simulink model "PR_2_var2"  (R2020b)
settings: Solver=VariableStepAuto  StartTime=0.0  StopTime=50  FixedStep=10^-4  RelTol=1e-3
libraries: simulink x2
settings Model: Creator=SIA  LastModifiedBy=SIA

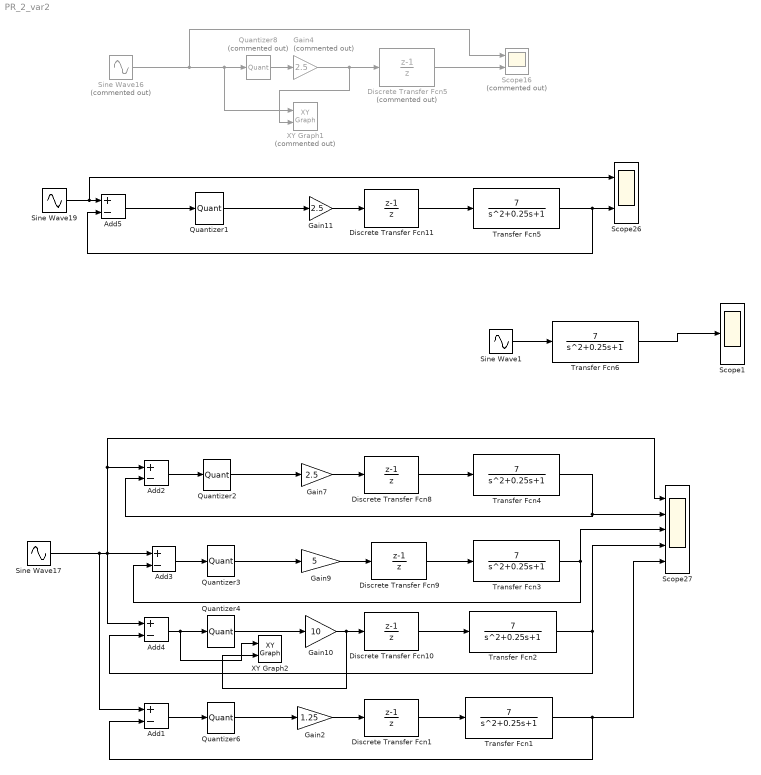
== system PR_2_var2 ==
  Add{1..5} (5 alike) : Sum  Inputs=+-
  Discrete Transfer Fcn{1,8..11} (5 alike) : DiscreteTransferFcn  Numerator=[1 -1]  Denominator=[1 0]  SampleTime=0.05
  Discrete Transfer Fcn5 : DiscreteTransferFcn  Commented=on  Numerator=[1 -1]  Denominator=[1 0]  SampleTime=0.05
  Gain10 : Gain  Gain=10
  Gain11 : Gain  Gain=2.5
  Gain2 : Gain  Gain=1.25
  Gain4 : Gain  Commented=on  Gain=2.5
  Gain7 : Gain  Gain=2.5
  Gain9 : Gain  Gain=5
  Quantizer1 : Quantizer  QuantizationInterval=2
  Quantizer2 : Quantizer  QuantizationInterval=2
  Quantizer3 : Quantizer  QuantizationInterval=1
  Quantizer4 : Quantizer
  Quantizer6 : Quantizer  QuantizationInterval=4
  Quantizer8 : Quantizer  Commented=on  QuantizationInterval=2
  Scope1 : Scope  NumInputPorts=3
  Scope16 : Scope  Commented=on  NumInputPorts=2
  Scope26 : Scope  NumInputPorts=2
  Scope27 : Scope  NumInputPorts=5
  Sine Wave1 : Sin  Amplitude=5*0.5  Frequency=3  SampleTime=0
  Sine Wave16 : Sin  Commented=on  Amplitude=5*1  SampleTime=0
  Sine Wave17 : Sin  Amplitude=5*1  SampleTime=0
  Sine Wave19 : Sin  Amplitude=5*1  SampleTime=0
  Transfer Fcn{1..6} (6 alike) : TransferFcn  Numerator=[7]  Denominator=[1 0.25 1]
  XY Graph1 : simulink/Sinks/XY Graph  Commented=on  xmin=-10  xmax=10  ymin=-15  ymax=15  st=-1
  XY Graph2 : simulink/Sinks/XY Graph  xmin=-5  xmax=5  ymin=-10  ymax=10  st=0.01
  wires:
  Quantizer8/1 -> Gain4/1
  Discrete Transfer Fcn5/1 -> Scope16/2
  Transfer Fcn5/1 -> Add5/2, Scope26/2
  Sine Wave19/1 -> Scope26/1, Add5/1
  Add5/1 -> Quantizer1/1
  Discrete Transfer Fcn11/1 -> Transfer Fcn5/1
  Gain11/1 -> Discrete Transfer Fcn11/1
  Quantizer2/1 -> Gain7/1
  Transfer Fcn4/1 -> Scope27/2, Add2/2
  Discrete Transfer Fcn8/1 -> Transfer Fcn4/1
  Add2/1 -> Quantizer2/1
  Gain7/1 -> Discrete Transfer Fcn8/1
  Quantizer3/1 -> Gain9/1
  Transfer Fcn3/1 -> Add3/2, Scope27/3
  Discrete Transfer Fcn9/1 -> Transfer Fcn3/1
  Add3/1 -> Quantizer3/1
  Gain9/1 -> Discrete Transfer Fcn9/1
  Quantizer4/1 -> Gain10/1
  Transfer Fcn2/1 -> Scope27/4, Add4/2
  Discrete Transfer Fcn10/1 -> Transfer Fcn2/1
  Add4/1 -> XY Graph2/1, Quantizer4/1
  Gain10/1 -> XY Graph2/2, Discrete Transfer Fcn10/1
  Quantizer1/1 -> Gain11/1
  Gain4/1 -> Discrete Transfer Fcn5/1, XY Graph1/2
  Sine Wave16/1 -> Scope16/1, XY Graph1/1, Quantizer8/1
  Transfer Fcn1/1 -> Scope27/5, Add1/2
  Quantizer6/1 -> Gain2/1
  Sine Wave17/1 -> Add1/1, Add2/1, Scope27/1, Add4/1, Add3/1
  Gain2/1 -> Discrete Transfer Fcn1/1
  Add1/1 -> Quantizer6/1
  Discrete Transfer Fcn1/1 -> Transfer Fcn1/1
  Sine Wave1/1 -> Transfer Fcn6/1
  Transfer Fcn6/1 -> Scope1/2
